simulink model "txline_filter"  (Simulink 6.0)
settings: Solver=ode45  StartTime=0.0  StopTime=10  RelTol=1e-3
undefined symbols (not defined in the file or in its folder): Fs
libraries: rftxlines1 x6, rfports1 x4, dspsnks4 x1, simulink x1, dspsrcs4 x1
settings Model: Creator=RobertZ  LastModifiedBy=rzeng  ProdHWDeviceType=Specified  UpdateModelReferenceTargets=IfOutOfDate
settings DataIOCC: SaveOutput=off  SaveTime=off  SignalLoggingName=sigsOut
settings DebuggingCC: CheckExecutionContextPreStartOutputMsg=on  CheckExecutionContextRuntimeOutputMsg=on  SolverPrmCheckMsg=none
settings HardwareCC: ProdHWDeviceType=Specified
settings ModelReferenceCC: UpdateModelReferenceTargets=IfOutOfDate
settings GRTTargetCC: UtilityFuncGeneration=Automatic  LifeSpan=inf
settings SFSimCC: SFSimApplyToAllLibs=on  SFSimBuildMode=Incremental

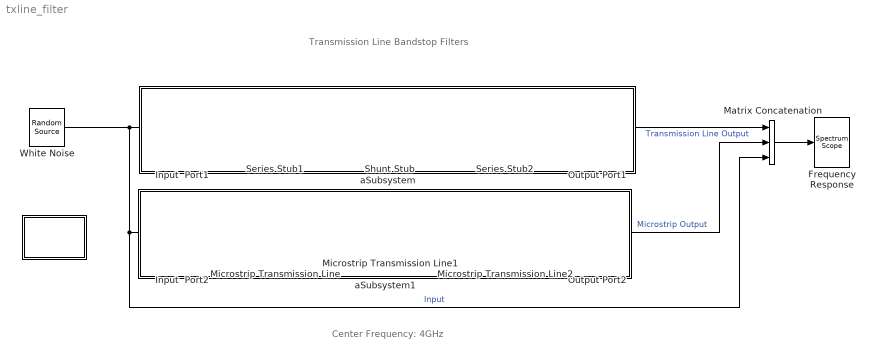
== system txline_filter ==
  note: Transmission Line Bandstop Filters
  note: Center Frequency: 4GHz
  " " : Subsystem  EnableExecutionContextPropagation=on
      mask Type: Interpolation filter info block
      mask Display: disp('Info')
  Frequency Response : dspsnks4/Spectrum Scope  ScopeProperties=off  Domain=Frequency  HorizSpan=1  UseBuffer=off  BufferSize=1024  Overlap=512  inpFftLenInherit=on  FFTlength=1024  numAvg=100  DisplayProperties=off  AxisGrid=on  Memory=off  FrameNumber=on  AxisLegend=on  AxisZoom=off  OpenScopeAtSimStart=on  OpenScopeImmediately=off  FigPos=[215 317 403 201]  AxisProperties=off  XUnits=Hertz  XRange=[-Fs/2...Fs/2]  InheritXIncr=off  XIncr=1/5e9  XLabel=Samples  YUnits=dB  YLabel=Magnitude, dB  LineProperties=on  LineColors='k'|'b'|'r'
      settings: YMin=-40  YMax=35
  Input  Port1 : rfports1/Input Port  Description=source block  MaxLength=128  Fc=4e9  Ts=1/5e9  Zs=50  NoiseFlag=off  seed=67987  GoToTag=ACBFHCICWIVGOQFZQMSDURJ
  Input  Port2 : rfports1/Input Port  Description=source block  MaxLength=128  Fc=4e9  Ts=1/5e9  Zs=50  NoiseFlag=off  seed=67987  GoToTag=BACGIDJDAJWHPAGARNTEVSK
  Matrix Concatenation : simulink/Math Operations/Matrix Concatenation  numInports=3  catMethod=Horizontal
  Microstrip Transmission Line : rftxlines1/Microstrip Transmission Line  PhysicalDomain=rfsystemsdomain  SubClassName=microstrip  LeftPortType=p1  RightPortType=p1  LConnTagsString=__newl0  RConnTagsString=__newr0  Width=2.6501e-3  Height=0.635e-3  Thickness=0.01e-3  EpsilonR=9.8  SigmaCond=inf  LossTangent=0  LineLength=0.00663  StubMode=Series  Termination=Short  DisplayData=off  PlotFreq=Derived from Input Port parameters  PlotFreqNoSim=User specified  Freq=1.5e9:10e6:6.5e9  AllPlotType=X-Y plane  NetworkData=S21  SmithData=S11  PolarData=S11  ComplexFormat=Magnitude (decibels)  DBFormat=Magnitude (decibels)  NoneFormat=None
  Microstrip Transmission Line1 : rftxlines1/Microstrip Transmission Line  PhysicalDomain=rfsystemsdomain  SubClassName=microstrip  LeftPortType=p1  RightPortType=p1  LConnTagsString=__newl0  RConnTagsString=__newr0  Width=0.40564e-3  Height=0.635e-3  Thickness=0.01e-3  EpsilonR=9.8  SigmaCond=inf  LossTangent=0  LineLength=0.00735  StubMode=Shunt  Termination=Open  DisplayData=off  PlotFreq=User specified  PlotFreqNoSim=User specified  Freq=1.5e9:10e6:6.5e9  AllPlotType=X-Y plane  NetworkData=S21  SmithData=S11  PolarData=S11  ComplexFormat=Magnitude (decibels)  DBFormat=Magnitude (decibels)  NoneFormat=None
  Microstrip Transmission Line2 : rftxlines1/Microstrip Transmission Line  PhysicalDomain=rfsystemsdomain  SubClassName=microstrip  LeftPortType=p1  RightPortType=p1  LConnTagsString=__newl0  RConnTagsString=__newr0  Width=2.6501e-3  Height=0.635e-3  Thickness=0.01e-3  EpsilonR=9.8  SigmaCond=inf  LossTangent=0  LineLength=0.00663  StubMode=Series  Termination=Short  DisplayData=off  PlotFreq=User specified  PlotFreqNoSim=User specified  Freq=1.5e9:10e6:6.5e9  AllPlotType=X-Y plane  NetworkData=S21  SmithData=S11  PolarData=S11  ComplexFormat=Magnitude (decibels)  DBFormat=Magnitude (decibels)  NoneFormat=None
  Output Port1 : rfports1/Output Port  Zl=50  num_Models=1  GoToTag=ACBFHCICWIVGOQFZQMSDURJ  DisplayData=off  PlotFreq=Derived from Input Port parameters  Freq=1e9:1e8:3e9  AllPlotType=Composite data  NoBudgetPlot=Composite data  NetworkData=S11  SmithData=S11  PolarData=S11  ComplexFormat=Magnitude (decibels)  DBFormat=Magnitude (decibels)  DBMFormat=dBm  NoneFormat=None
  Output Port2 : rfports1/Output Port  Zl=50  num_Models=1  GoToTag=BACGIDJDAJWHPAGARNTEVSK  DisplayData=off  PlotFreq=Derived from Input Port parameters  Freq=1e9:1e8:3e9  AllPlotType=Composite data  NoBudgetPlot=Composite data  NetworkData=S11  SmithData=S11  PolarData=S11  ComplexFormat=Magnitude (decibels)  DBFormat=Magnitude (decibels)  DBMFormat=dBm  NoneFormat=None
  Series Stub1 : rftxlines1/Transmission Line  PhysicalDomain=rfsystemsdomain  SubClassName=txline  LeftPortType=p1  RightPortType=p1  LConnTagsString=__newl0  RConnTagsString=__newr0  Z0=20.71  PV=1.8e8  Loss=0  LineLength=0.0113  StubMode=Series  Termination=Short  DisplayData=off  PlotFreq=User specified  PlotFreqNoSim=User specified  Freq=1.5e9:10e6:6.5e9  AllPlotType=X-Y plane  NetworkData=S21  SmithData=S11  PolarData=S11  ComplexFormat=Magnitude (decibels)  DBFormat=Magnitude (decibels)  NoneFormat=None
  Series Stub2 : rftxlines1/Transmission Line  PhysicalDomain=rfsystemsdomain  SubClassName=txline  LeftPortType=p1  RightPortType=p1  LConnTagsString=__newl0  RConnTagsString=__newr0  Z0=20.71  PV=1.8e8  Loss=0  LineLength=0.0113  StubMode=Series  Termination=Short  DisplayData=off  PlotFreq=Derived from Input Port parameters  PlotFreqNoSim=User specified  Freq=1.5e9:10e6:6.5e9  AllPlotType=X-Y plane  NetworkData=S21  SmithData=S11  PolarData=S11  ComplexFormat=Magnitude (decibels)  DBFormat=Magnitude (decibels)  NoneFormat=None
  Shunt Stub : rftxlines1/Transmission Line  PhysicalDomain=rfsystemsdomain  SubClassName=txline  LeftPortType=p1  RightPortType=p1  LConnTagsString=__newl0  RConnTagsString=__newr0  Z0=60.355  PV=1.8e8  Loss=0  LineLength=0.0113  StubMode=Shunt  Termination=Open  DisplayData=off  PlotFreq=Derived from Input Port parameters  PlotFreqNoSim=User specified  Freq=1.5e9:10e6:6.5e9  AllPlotType=X-Y plane  NetworkData=S21  SmithData=S11  PolarData=S11  ComplexFormat=Magnitude (decibels)  DBFormat=Magnitude (decibels)  NoneFormat=None
  White Noise : dspsrcs4/Random Source  SrcType=Gaussian  NormMethod=Ziggurat  CltLength=12  Min=-1.25  Max=1.25  Mean=0  Var=1  RepMode=Not repeatable  Seed=1  Inherit=off  SampMode=Discrete  SampTime=1/5e9  SampFrame=256  DataType=Double  OutComplex=Complex
  aSubsystem : Subsystem  EnableExecutionContextPropagation=on
      mask Display: disp('')
  aSubsystem1 : Subsystem  EnableExecutionContextPropagation=on
      mask Display: disp('')
  wires:
  White Noise/1 -> Input  Port1/1, Matrix Concatenation/3, Input  Port2/1  "Input"
  Matrix Concatenation/1 -> Frequency Response/1
  Output Port1/1 -> Matrix Concatenation/1  "Transmission Line Output"
  Output Port2/1 -> Matrix Concatenation/2  "Microstrip Output"
  connections:
  Series Stub1/LConn1 -- Input  Port1/RConn1
  Series Stub1/RConn1 -- Shunt Stub/LConn1
  Shunt Stub/RConn1 -- Series Stub2/LConn1
  Series Stub2/RConn1 -- Output Port1/LConn1
  Input  Port2/RConn1 -- Microstrip Transmission Line/LConn1
  Microstrip Transmission Line/RConn1 -- Microstrip Transmission Line1/LConn1
  Microstrip Transmission Line1/RConn1 -- Microstrip Transmission Line2/LConn1
  Microstrip Transmission Line2/RConn1 -- Output Port2/LConn1

== system txline_filter/  ==
  note: Transmission Line Bandstop Filters
      |
      | The RF Blockset has the following blocks for transmission lines:
      | Coaxial Transmission Line
      | Transmission Line
      | Microstrip Transmission Line
      | Parallel Plate Transmission Line
      | Two Wire Transmission Line
      | Coplanar Waveguide Transmission Line
      |
      | This demo simulates a bandstop Transmission Line filter and
      | a bandstop Microstrip filter with a Gaussian random signal input.
      |
      | The spectrum plot shows frequency ranging from
      | 1.5GHz to 6.5GHz centered at 4GHz.
      |
      |
      | If you want to see the frequency response centered at other RF frequency,
      | you need to change the Center frequency parameter in the
      | 'Input Port' block.
      |
      | If you want to change the range of frequency response that is determined by
      | the Sample time parameter specified in the 'Input Port' and 'White Noise' blocks,
      | you need to change the Sample time parameter in both blocks.

== system txline_filter/aSubsystem ==

== system txline_filter/aSubsystem1 ==
